simulink model "Pacing"  (R2022b)
settings: Solver=FixedStepAuto  StartTime=0.0  StopTime=10.0  FixedStep=1e-3  RelTol=1e-3  EnableMultiTasking=on
undefined symbols (not defined in the file): A0, A1, PTB2, PTB3
libraries: frdmk64flib x5, etargetslib x3
settings Model: ExtModeTrigDuration=5  Creator=Ali Umar  LastModifiedBy=seankhaira
settings OptimizationCC: EnhancedBackFolding=on  PassReuseOutputArgsAs=Individual arguments  ZeroExternalMemoryAtStartup=off  ZeroInternalMemoryAtStartup=off  MaxStackSize=64  OptimizeBlockOrder=speed  DifferentSizesBufferReuse=on  OptimizationCustomize=off  EfficientTunableParamExpr=on
settings DebuggingCC: ParameterTunabilityLossMsg=error
settings HardwareCC: ProdBitPerPointer=32  ProdBitPerSizeT=32  ProdBitPerPtrDiffT=32  ProdLargestAtomicInteger=Long  ProdLargestAtomicFloat=Double  ProdWordSize=32  ProdHWDeviceType=ARM Compatible->ARM Cortex
settings SFSimCC: MATLABDynamicMemAlloc=off
settings RTWCC: Description=Embedded Coder  SystemTargetFile=ert.tlc  HardwareBoard=NXP FRDM-K64F  TLCOptions="-aInlineSetEventsForThisBaseRateFcn=TLC_FALSE -aSuppressMultiTaskScheduler=TLC_FALSE  -aRateBasedStepFcn=0"  TemplateMakefile=ert_default_tmf  Toolchain=GNU Tools for ARM Embedded Processors
settings CodeAppCC: ForceParamTrailComments=on  IgnoreCustomStorageClasses=off  OperatorAnnotations=on  SimulinkDataObjDesc=on  SFDataObjDesc=on  InsertBlockDesc=on
settings ERTTargetCC: ExtModeTransport=4  ExtModeMexFile=sendToCommService

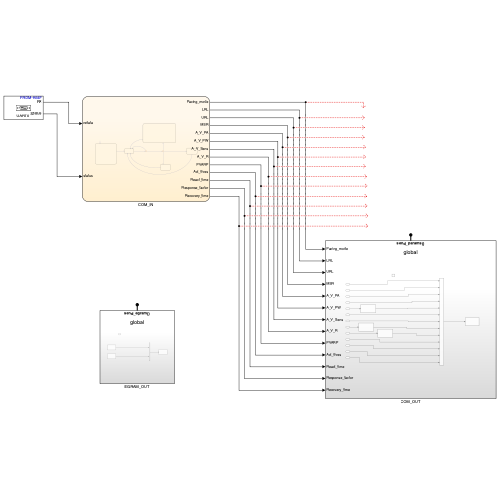
[thumbnail: Simulink's stored preview of the top-level diagram]
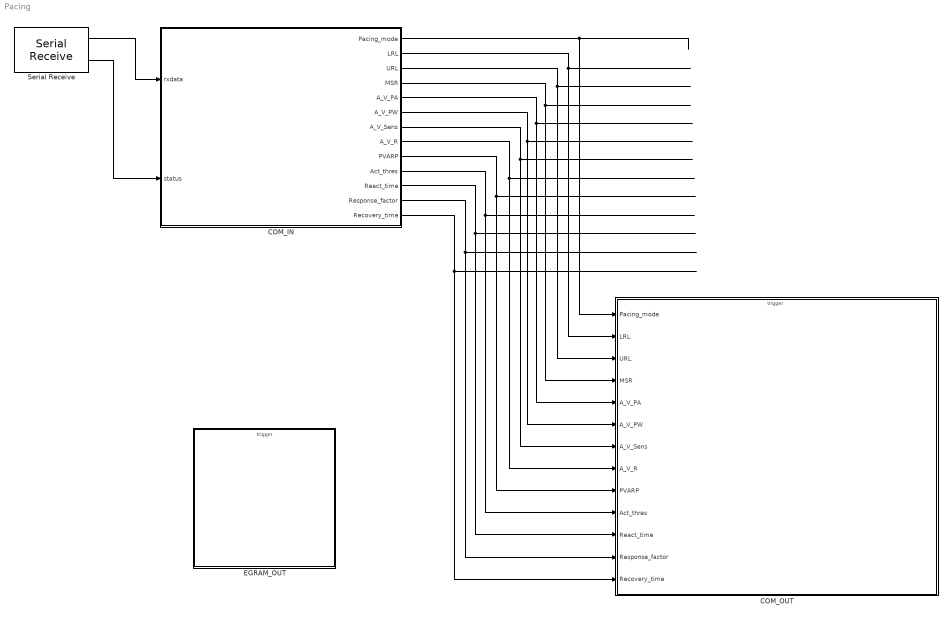
== system Pacing ==
  COM_IN : Stateflow chart  TreatAsAtomicUnit=on
  COM_OUT : Subsystem  TreatAsAtomicUnit=on
  EGRAM_OUT : Subsystem  TreatAsAtomicUnit=on
  Serial Receive : frdmk64flib/Serial Receive  SCIModule=0  Baudrate=uint32(9600)  Parity=None  StopBits=1  HardwareFlowControl=None  ByteOrder=LittleEndian  DataType=uint8  DataLength=6  BlockingMode=off  OutputStatus=on  SampleTime=-1
  wires:
  Serial Receive/2 -> COM_IN/2(status)
  Serial Receive/1 -> COM_IN/1(rxdata)
  COM_IN/1(Pacing_mode) -> COM_OUT/1(Pacing_mode)
  COM_IN/2(LRL) -> COM_OUT/2(LRL)
  COM_IN/3(URL) -> COM_OUT/3(URL)
  COM_IN/4(MSR) -> COM_OUT/4(MSR)
  COM_IN/5(A_V_PA) -> COM_OUT/5(A_V_PA)
  COM_IN/6(A_V_PW) -> COM_OUT/6(A_V_PW)
  COM_IN/7(A_V_Sens) -> COM_OUT/7(A_V_Sens)
  COM_IN/8(A_V_R) -> COM_OUT/8(A_V_R)
  COM_IN/9(PVARP) -> COM_OUT/9(PVARP)
  COM_IN/10(Act_thres) -> COM_OUT/10(Act_thres)
  COM_IN/11(React_time) -> COM_OUT/11(React_time)
  COM_IN/12(Response_factor) -> COM_OUT/12(Response_factor)
  COM_IN/13(Recovery_time) -> COM_OUT/13(Recovery_time)

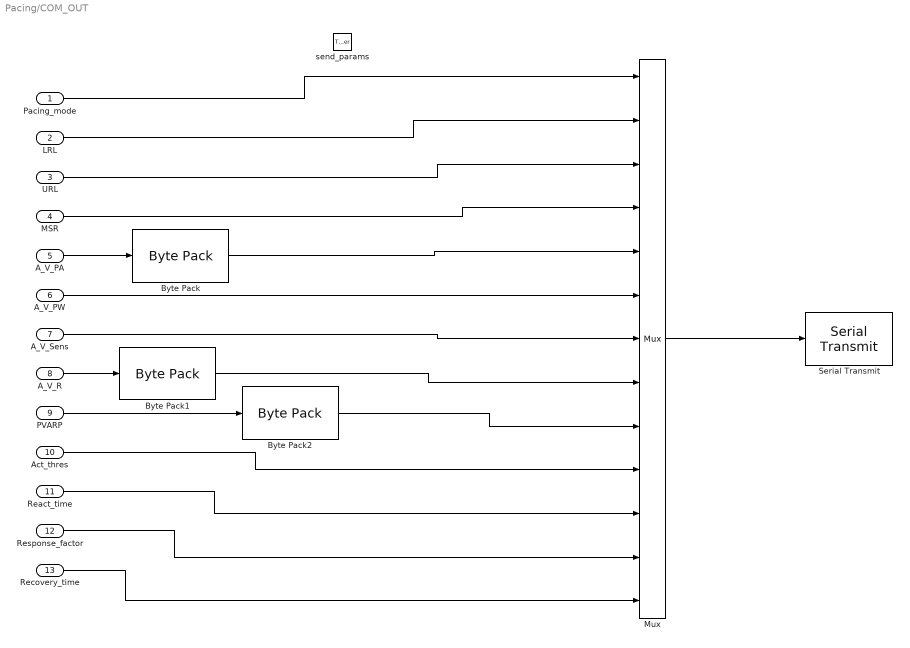
== system Pacing/COM_OUT ==
  Pacing_mode : Inport
  LRL : Inport  Port=2
  URL : Inport  Port=3
  MSR : Inport  Port=4
  A_V_PA : Inport  Port=5
  A_V_PW : Inport  Port=6
  A_V_Sens : Inport  Port=7
  A_V_R : Inport  Port=8
  PVARP : Inport  Port=9
  Act_thres : Inport  Port=10
  React_time : Inport  Port=11
  Response_factor : Inport  Port=12
  Recovery_time : Inport  Port=13
  send_params : TriggerPort  TriggerType=function-call  IsSimulinkFunction=on  FunctionName=send_params  VariantControl=(inherit)
  Byte Pack : etargetslib/Byte Pack  datatypes={'single'}  byteAlign=1
  Byte Pack1 : etargetslib/Byte Pack  datatypes={'uint16'}  byteAlign=1
  Byte Pack2 : etargetslib/Byte Pack  datatypes={'uint16'}  byteAlign=1
  Mux : Mux  Inputs=13
  Serial Transmit : frdmk64flib/Serial Transmit  SCIModule=0  Baudrate=uint32(9600)  Parity=None  StopBits=1  HardwareFlowControl=None  ByteOrder=LittleEndian  BlockingMode=on  OutputStatus=off
  wires:
  Mux/1 -> Serial Transmit/1
  Pacing_mode/1 -> Mux/1
  LRL/1 -> Mux/2
  URL/1 -> Mux/3
  MSR/1 -> Mux/4
  A_V_PW/1 -> Mux/6
  A_V_Sens/1 -> Mux/7
  Act_thres/1 -> Mux/10
  React_time/1 -> Mux/11
  Response_factor/1 -> Mux/12
  Recovery_time/1 -> Mux/13
  A_V_PA/1 -> Byte Pack/1
  Byte Pack/1 -> Mux/5
  A_V_R/1 -> Byte Pack1/1
  Byte Pack1/1 -> Mux/8
  PVARP/1 -> Byte Pack2/1
  Byte Pack2/1 -> Mux/9

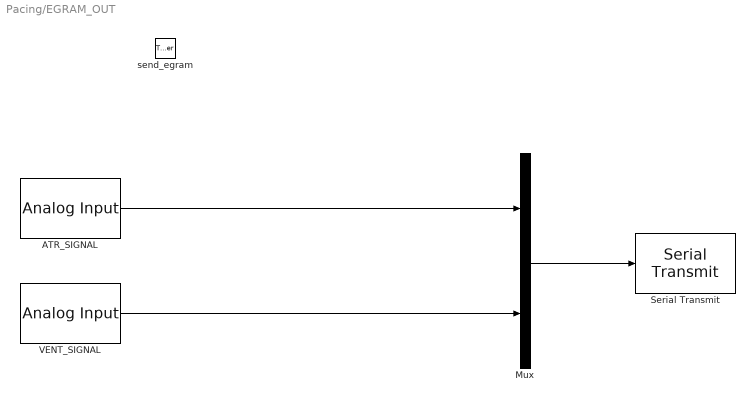
== system Pacing/EGRAM_OUT ==
  send_egram : TriggerPort  TriggerType=function-call  IsSimulinkFunction=on  FunctionName=send_egram  VariantControl=(inherit)
  ATR_SIGNAL : frdmk64flib/Analog Input  Whichpin=PTB2 (A0)  SampleTime=-1
  Mux : Mux  Inputs=2
  Serial Transmit : frdmk64flib/Serial Transmit  SCIModule=0  Baudrate=uint32(9600)  Parity=None  StopBits=1  HardwareFlowControl=None  ByteOrder=LittleEndian  BlockingMode=on  OutputStatus=off
  VENT_SIGNAL : frdmk64flib/Analog Input  Whichpin=PTB3 (A1)  SampleTime=-1
  wires:
  ATR_SIGNAL/1 -> Mux/1
  VENT_SIGNAL/1 -> Mux/2
  Mux/1 -> Serial Transmit/1

== stateflow chart Pacing/COM_IN ==
  settings: executeAtInitialization=1
  state SET_PARAM
    entry:
    Pacing_mode = rxdata(3);%1-8
    LRL = rxdata(4);%ppm
    URL = rxdata(5);%ppm
    MSR = rxdata(6);%max sensor rate ppm
    A_V_PA = typecast(rxdata(7:10), 'single');%pulse amplitude V
    A_V_PW = rxdata(11);%ms
    A_V_Sens = rxdata(12);%sensitivity V
    A_V_R = typecast(rxdata(13:14), 'uint16');%refractory ms
    PVARP = typecast(rxdata(15:16), 'uint16');%ms
    Act_thres = rxdata(17);%7 levels
    React_time = rxdata(18);%sec
    Response_factor = rxdata(19);%16 levels
    Recovery_time = rxdata(20);%mins
  state INITIAL
    %set initial parameters
    entry:
    Pacing_mode = 1;%1-8
    LRL = 50;%ppm
    URL = 50;%ppm
    MSR = 50;%max sensor rate ppm
    A_V_PA = 0.0;%pulse amplitude V
    A_V_PW = 1;%ms
    A_V_Sens = 0;%sensitivity V
    A_V_R = 150;%refractory ms
    PVARP = 150;%ms
    Act_thres = 1;%7 levels
    React_time = 10;%sec
    Response_factor = 1;%16 levels
    Recovery_time = 2;%mins
  state EGRAM
    entry:
    send_egram();
  state STANDBY
    %wait for com
  state ECHO_PARAM
    entry:
    send_params();
  SET_PARAM -> STANDBY
  (default) -> INITIAL
  (junction 21) -> SET_PARAM [order 1] : [rxdata(2)== hex2dec('55')]
  (junction 18) -> STANDBY [order 2]
  INITIAL -> STANDBY
  STANDBY -> (junction 18) : [status==0]
  (junction 18) -> (junction 21) [order 1] : [rxdata(1)== hex2dec('16')]
  (junction 21) -> EGRAM [order 3] : [rxdata(2)== hex2dec('61')]
  (junction 21) -> ECHO_PARAM [order 2] : [rxdata(2)== hex2dec('22')]
  EGRAM -> STANDBY
  ECHO_PARAM -> STANDBY
  data: rxdata input; status input; Pacing_mode output uint8; LRL output uint8; URL output uint8; MSR output uint8; A_V_PA output; A_V_PW output; A_V_Sens output; A_V_R output; PVARP output; Act_thres output; React_time output; Response_factor output; Recovery_time output
